simulink model "Disconnections_ETR07"  (R2017b)
settings: Solver=FixedStepAuto  StartTime=0.0  StopTime=10.0  RelTol=1e-3
libraries: simulink x7
settings Model: Creator=cspt  LastModifiedBy=cspt
settings RTWCC: SystemTargetFile=irt.tlc  TemplateMakefile=irt_default_tmf  Description=INTECRIO Real-Time Target
settings STFCustomTargetCC: TargetLangStandard=C99 (ISO)  UtilityFuncGeneration=Shared location  SystemTargetFile=irt.tlc
settings GRTTargetCC: UtilityFuncGeneration=Shared location  ParMdlRefBuildCompliant=off  CompOptLevelCompliant=off  ConcurrentExecutionCompliant=off  CombineOutputUpdateFcns=off  MatFileLogging=off  CPPClassGenCompliant=off  GRTInterface=on  UseToolchainInfoCompliant=off  GenerateASAP2=on

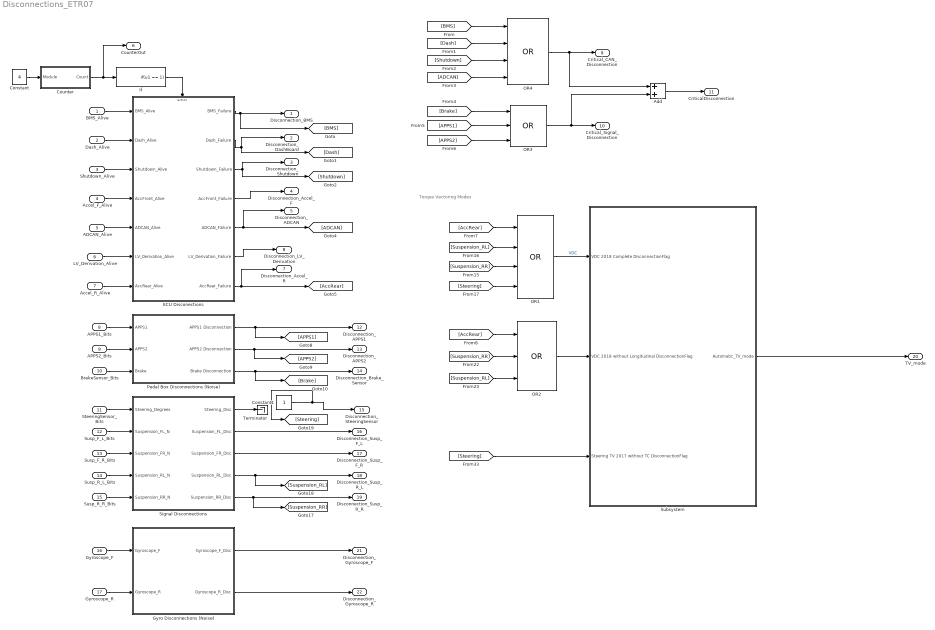
== system Disconnections_ETR07 ==
  note: Torque Vectoring Modes
  BMS_Alive : Inport
  Dash_Alive : Inport  Port=2
  Shutdown_Alive : Inport  Port=3
  Accel_F_Alive : Inport  Port=4
  ADCAN_Alive : Inport  Port=5
  LV_Derivation_Alive : Inport  Port=6
  Accel_R_Alive : Inport  Port=7
  APPS1_Bits : Inport  Port=8
  APPS2_Bits : Inport  Port=9
  BrakeSensor_Bits : Inport  Port=10
  SteeringSensor_Bits : Inport  Port=11
  Susp_F_L_Bits : Inport  Port=12
  Susp_F_R_Bits : Inport  Port=13
  Susp_R_L_Bits : Inport  Port=14
  Susp_R_R_Bits : Inport  Port=15
  Gyroscope_F : Inport  Port=16
  Gyroscope_R : Inport  Port=17
  Add : Sum
  Constant : Constant  Value=4
  Constant1 : Constant
  Counter : Subsystem
  ECU Disconections : Subsystem
  Gyro Disconnections (Noise) : Subsystem
  If : If  IfExpression=u1 == 1  ShowElse=off
  OR1 : Logic  Operator=OR  Inputs=4  AllPortsSameDT=off  OutDataTypeStr=boolean
  OR2 : Logic  Operator=OR  Inputs=3  AllPortsSameDT=off  OutDataTypeStr=boolean
  OR3 : Logic  Operator=OR  Inputs=3  AllPortsSameDT=off  OutDataTypeStr=boolean
  OR4 : Logic  Operator=OR  Inputs=4  AllPortsSameDT=off  OutDataTypeStr=boolean
  Pedal Box Disconnections (Noise) : Subsystem
  Signal Disconnections : Subsystem
  Subsystem : Subsystem
  Terminator : Terminator
  Disconnection_BMS : Outport
  Disconnection_DashBoard : Outport  Port=2
  Disconnection_Shutdown : Outport  Port=3
  Disconnection_Accel_F : Outport  Port=4
  Disconnection_ADCAN : Outport  Port=5
  CounterOut : Outport  Port=6
  Disconnection_Accel_R : Outport  Port=7
  Disconnection_LV_Derivation : Outport  Port=8
  Critical_CAN_Disconnection : Outport  Port=9
  Critical_Signal_Disconnection : Outport  Port=10
  CriticalDisconnection : Outport  Port=11
  Disconnection_APPS1 : Outport  Port=12
  Disconnection_APPS2 : Outport  Port=13
  Disconnection_Brake_Sensor : Outport  Port=14
  Disconnection_SteeringSensor : Outport  Port=15
  Disconnection_Susp_F_L : Outport  Port=16
  Disconnection_Susp_F_R : Outport  Port=17
  Disconnection_Susp_R_L : Outport  Port=18
  Disconnection_Susp_R_R : Outport  Port=19
  TV_mode : Outport  Port=20
  Disconnection_Gyroscope_F : Outport  Port=21
  Disconnection_Gyroscope_R : Outport  Port=22
  wires:
  LV_Derivation_Alive/1 -> ECU Disconections/6(LV_Derivation_Alive)
  Accel_R_Alive/1 -> ECU Disconections/7(AccRear_Alive)
  ECU Disconections/7(AccRear_Failure) -> [AccRear], Disconnection_Accel_R/1
  ECU Disconections/5(ADCAN_Failure) -> Disconnection_ADCAN/1, [ADCAN]
  ECU Disconections/1(BMS_Failure) -> Disconnection_BMS/1, [BMS]
  Dash_Alive/1 -> ECU Disconections/2(Dash_Alive)
  ECU Disconections/4(AccFront_Failure) -> Disconnection_Accel_F/1
  Counter/1(Count) -> CounterOut/1, If/1
  ECU Disconections/6(LV_Derivation_Failure) -> Disconnection_LV_Derivation/1
  Accel_F_Alive/1 -> ECU Disconections/4(AccFront_Alive)
  BMS_Alive/1 -> ECU Disconections/1(BMS_Alive)
  Constant/1 -> Counter/1(Module)
  ECU Disconections/2(Dash_Failure) -> Disconnection_DashBoard/1, [Dash]
  Shutdown_Alive/1 -> ECU Disconections/3(Shutdown_Alive)
  If/1 -> ECU Disconections/Action
  ECU Disconections/3(Shutdown_Failure) -> [Shutdown], Disconnection_Shutdown/1
  ADCAN_Alive/1 -> ECU Disconections/5(ADCAN_Alive)
  [Shutdown] -> OR4/3
  [Dash] -> OR4/2
  [BMS] -> OR4/1
  [ADCAN] -> OR4/4
  [Brake] -> OR3/1
  [APPS1] -> OR3/2
  OR3/1 -> Add/2, Critical_Signal_Disconnection/1
  [APPS2] -> OR3/3
  Add/1 -> CriticalDisconnection/1
  OR4/1 -> Add/1, Critical_CAN_Disconnection/1
  Pedal Box Disconnections (Noise)/2(APPS2 Disconnection) -> Disconnection_APPS2/1, [APPS2]
  Pedal Box Disconnections (Noise)/3(Brake Disconnection) -> Disconnection_Brake_Sensor/1, [Brake]
  APPS2_Bits/1 -> Pedal Box Disconnections (Noise)/2(APPS2)
  BrakeSensor_Bits/1 -> Pedal Box Disconnections (Noise)/3(Brake)
  Pedal Box Disconnections (Noise)/1(APPS1 Disconnection) -> [APPS1], Disconnection_APPS1/1
  APPS1_Bits/1 -> Pedal Box Disconnections (Noise)/1(APPS1)
  Signal Disconnections/2(Suspension_FL_Disc) -> Disconnection_Susp_F_L/1
  Susp_R_L_Bits/1 -> Signal Disconnections/4(Suspension_RL_N)
  Signal Disconnections/4(Suspension_RL_Disc) -> Disconnection_Susp_R_L/1, [Suspension_RL]
  Signal Disconnections/5(Suspension_RR_Disc) -> Disconnection_Susp_R_R/1, [Suspension_RR]
  Susp_R_R_Bits/1 -> Signal Disconnections/5(Suspension_RR_N)
  Signal Disconnections/3(Suspension_FR_Disc) -> Disconnection_Susp_F_R/1
  Susp_F_R_Bits/1 -> Signal Disconnections/3(Suspension_FR_N)
  Susp_F_L_Bits/1 -> Signal Disconnections/2(Suspension_FL_N)
  SteeringSensor_Bits/1 -> Signal Disconnections/1(Steering_Degrees)
  [Steering] -> Subsystem/3(Steering TV 2017 without TC DisconnectionFlag)
  OR1/1 -> Subsystem/1(VDC 2018 Complete DisconnectionFlag)  "VDC"
  [Suspension_RR] -> OR2/2
  OR2/1 -> Subsystem/2(VDC 2018 without Longitudinal DisconnectionFlag)
  Subsystem/1(Automatic_TV_mode) -> TV_mode/1
  [Suspension_RL] -> OR2/3
  [AccRear] -> OR2/1
  [AccRear] -> OR1/1
  Gyro Disconnections (Noise)/2(Gyroscope_R_Disc) -> Disconnection_Gyroscope_R/1
  Gyro Disconnections (Noise)/1(Gyroscope_F_Disc) -> Disconnection_Gyroscope_F/1
  Gyroscope_R/1 -> Gyro Disconnections (Noise)/2(Gyroscope_R)
  Gyroscope_F/1 -> Gyro Disconnections (Noise)/1(Gyroscope_F)
  [Suspension_RL] -> OR1/2
  [Suspension_RR] -> OR1/3
  [Steering] -> OR1/4
  Signal Disconnections/1(Steering_Disc) -> Terminator/1
  Constant1/1 -> [Steering], Disconnection_SteeringSensor/1

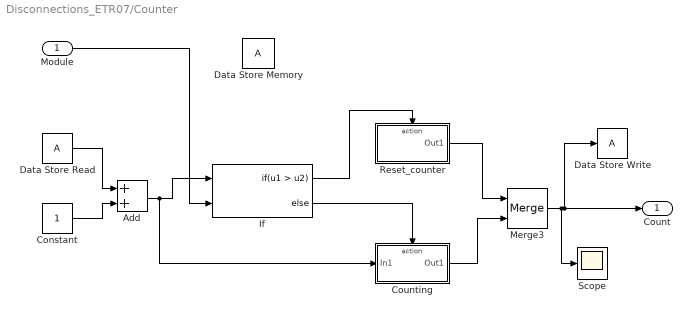
== system Disconnections_ETR07/Counter ==
  Module : Inport
  Add : Sum
  Constant : Constant
  Counting : Subsystem  TreatAsAtomicUnit=on
  Data Store Memory : DataStoreMemory  ReadBeforeWriteMsg=warning  WriteAfterWriteMsg=warning  WriteAfterReadMsg=warning  ShowAdditionalParam=off
  Data Store Read : DataStoreRead
  Data Store Write : DataStoreWrite
  If : If  NumInputs=2  IfExpression=u1 > u2
  Merge3 : Merge
  Reset_counter : Subsystem  TreatAsAtomicUnit=on
  Scope : Scope
  Count : Outport
  wires:
  Data Store Read/1 -> Add/1
  Constant/1 -> Add/2
  Add/1 -> If/1, Counting/1(In1)
  If/1 -> Reset_counter/Action
  If/2 -> Counting/Action
  Reset_counter/1(Out1) -> Merge3/1
  Counting/1(Out1) -> Merge3/2
  Module/1 -> If/2
  Merge3/1 -> Scope/1, Data Store Write/1, Count/1

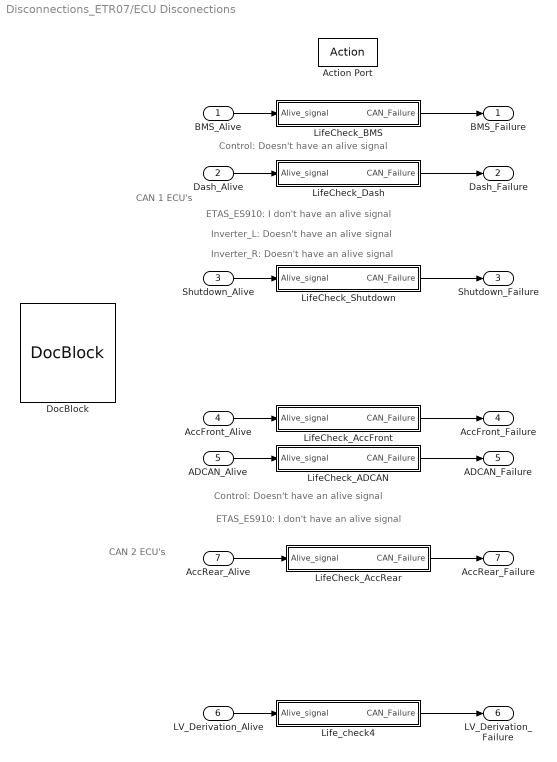
== system Disconnections_ETR07/ECU Disconections ==
  note: ETAS_ES910: I don't have an alive signal
  note: Control: Doesn't have an alive signal
  note: CAN 1
      | ECU's
  note: Inverter_L: Doesn't have an alive signal
  note: Inverter_R: Doesn't have an alive signal
  note: Control: Doesn't have an alive signal
  note: ETAS_ES910: I don't have an alive signal
  note: CAN 2
      | ECU's
  BMS_Alive : Inport
  Dash_Alive : Inport  Port=2
  Shutdown_Alive : Inport  Port=3
  AccFront_Alive : Inport  Port=4
  ADCAN_Alive : Inport  Port=5
  LV_Derivation_Alive : Inport  Port=6
  AccRear_Alive : Inport  Port=7
  Action Port : ActionPort  ActionType=then
  DocBlock : simulink/Model-Wide Utilities/DocBlock  DocumentType=Text
      content=|
      | The Alive signal is sent and updated every 4 synchronisms (25ms x 4 = 100ms).
      |
      | This is a Network Management Module. It takes all the alive signals of the ECU's and check if they are "alive".
      | All the ECU's for each CAN database have been extracted and listed. Some ECU's do not have an alive signal.
      |
      | Each LifeCheck generates a signal that indicate if the ECU has been disconnected.
      | OK -> 0
      | Disconnected -> 1
  LifeCheck_ADCAN : Subsystem
  LifeCheck_AccFront : Subsystem
  LifeCheck_AccRear : Subsystem
  LifeCheck_BMS : Subsystem
  LifeCheck_Dash : Subsystem
  LifeCheck_Shutdown : Subsystem
  Life_check4 : Subsystem
  BMS_Failure : Outport
  Dash_Failure : Outport  Port=2
  Shutdown_Failure : Outport  Port=3
  AccFront_Failure : Outport  Port=4
  ADCAN_Failure : Outport  Port=5
  LV_Derivation_Failure : Outport  Port=6
  AccRear_Failure : Outport  Port=7
  wires:
  Life_check4/1(CAN_Failure) -> LV_Derivation_Failure/1
  LV_Derivation_Alive/1 -> Life_check4/1(Alive_signal)
  LifeCheck_AccFront/1(CAN_Failure) -> AccFront_Failure/1
  LifeCheck_Shutdown/1(CAN_Failure) -> Shutdown_Failure/1
  LifeCheck_Dash/1(CAN_Failure) -> Dash_Failure/1
  Dash_Alive/1 -> LifeCheck_Dash/1(Alive_signal)
  LifeCheck_ADCAN/1(CAN_Failure) -> ADCAN_Failure/1
  LifeCheck_BMS/1(CAN_Failure) -> BMS_Failure/1
  AccFront_Alive/1 -> LifeCheck_AccFront/1(Alive_signal)
  BMS_Alive/1 -> LifeCheck_BMS/1(Alive_signal)
  ADCAN_Alive/1 -> LifeCheck_ADCAN/1(Alive_signal)
  Shutdown_Alive/1 -> LifeCheck_Shutdown/1(Alive_signal)
  LifeCheck_AccRear/1(CAN_Failure) -> AccRear_Failure/1
  AccRear_Alive/1 -> LifeCheck_AccRear/1(Alive_signal)

== system Disconnections_ETR07/Gyro Disconnections (Noise) ==
  Gyroscope_F : Inport
  Gyroscope_R : Inport  Port=2
  Life_check6 : Subsystem
  Life_check8 : Subsystem
  Gyroscope_F_Disc : Outport
  Gyroscope_R_Disc : Outport  Port=2
  wires:
  Gyroscope_F/1 -> Life_check6/1(Signal)
  Life_check8/1(Disconnect_Fail) -> Gyroscope_R_Disc/1
  Gyroscope_R/1 -> Life_check8/1(Signal)
  Life_check6/1(Disconnect_Fail) -> Gyroscope_F_Disc/1

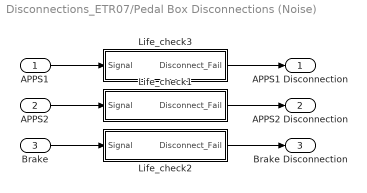
== system Disconnections_ETR07/Pedal Box Disconnections (Noise) ==
  APPS1 : Inport
  APPS2 : Inport  Port=2
  Brake : Inport  Port=3
  Life_check1 : Subsystem
  Life_check2 : Subsystem
  Life_check3 : Subsystem
  APPS1 Disconnection : Outport
  APPS2 Disconnection : Outport  Port=2
  Brake Disconnection : Outport  Port=3
  wires:
  Brake/1 -> Life_check2/1(Signal)
  APPS2/1 -> Life_check1/1(Signal)
  APPS1/1 -> Life_check3/1(Signal)
  Life_check3/1(Disconnect_Fail) -> APPS1 Disconnection/1
  Life_check1/1(Disconnect_Fail) -> APPS2 Disconnection/1
  Life_check2/1(Disconnect_Fail) -> Brake Disconnection/1

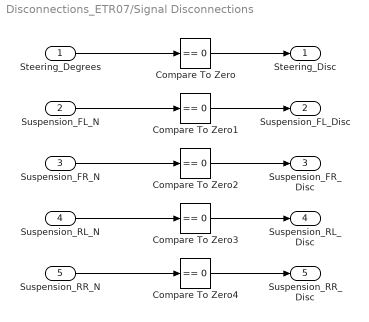
== system Disconnections_ETR07/Signal Disconnections ==
  Steering_Degrees : Inport
  Suspension_FL_N : Inport  Port=2
  Suspension_FR_N : Inport  Port=3
  Suspension_RL_N : Inport  Port=4
  Suspension_RR_N : Inport  Port=5
  Compare To Zero{,1..4} (5 alike) : simulink/Logic and Bit Operations/Compare To Zero  relop===  OutDataTypeStr=uint8
  Steering_Disc : Outport
  Suspension_FL_Disc : Outport  Port=2
  Suspension_FR_Disc : Outport  Port=3
  Suspension_RL_Disc : Outport  Port=4
  Suspension_RR_Disc : Outport  Port=5
  wires:
  Compare To Zero2/1 -> Suspension_FR_Disc/1
  Suspension_FR_N/1 -> Compare To Zero2/1
  Compare To Zero3/1 -> Suspension_RL_Disc/1
  Compare To Zero1/1 -> Suspension_FL_Disc/1
  Suspension_RR_N/1 -> Compare To Zero4/1
  Suspension_FL_N/1 -> Compare To Zero1/1
  Suspension_RL_N/1 -> Compare To Zero3/1
  Compare To Zero/1 -> Steering_Disc/1
  Steering_Degrees/1 -> Compare To Zero/1
  Compare To Zero4/1 -> Suspension_RR_Disc/1

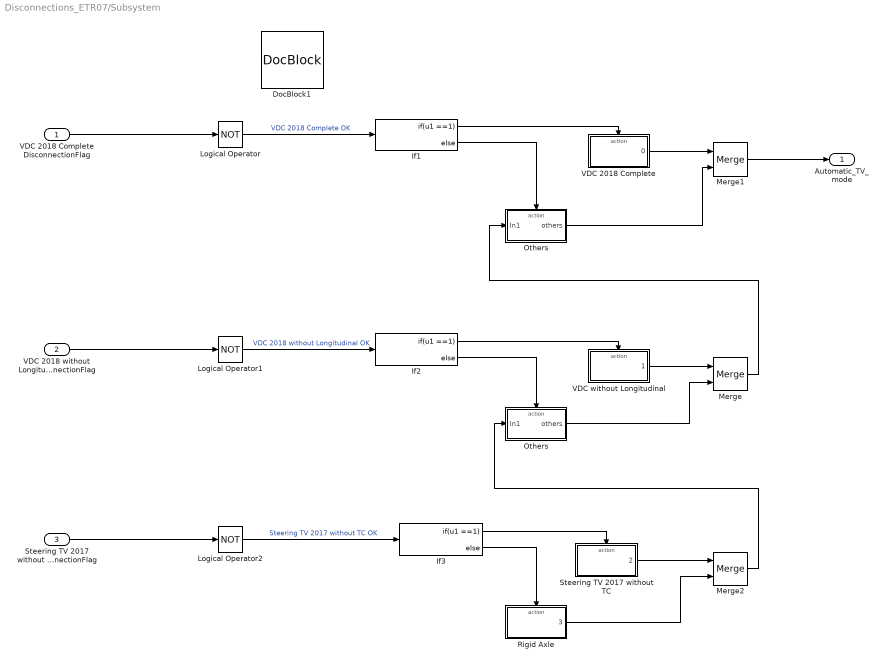
== system Disconnections_ETR07/Subsystem ==
  VDC 2018 Complete DisconnectionFlag : Inport
  VDC 2018 without Longitudinal DisconnectionFlag : Inport  Port=2
  Steering TV 2017 without TC DisconnectionFlag : Inport  Port=3
  DocBlock1 : simulink/Model-Wide Utilities/DocBlock  DocumentType=Text
      content=|
      | Checking for APPS, Brake etc... would be redundant since they are critical disconnections and the car will enter to a stop state
  If1 : If  IfExpression=u1 ==1
  If2 : If  IfExpression=u1 ==1
  If3 : If  IfExpression=u1 ==1
  Logical Operator : Logic  Operator=NOT  AllPortsSameDT=off  OutDataTypeStr=boolean
  Logical Operator1 : Logic  Operator=NOT  AllPortsSameDT=off  OutDataTypeStr=boolean
  Logical Operator2 : Logic  Operator=NOT  AllPortsSameDT=off  OutDataTypeStr=boolean
  Merge : Merge
  Merge1 : Merge
  Merge2 : Merge
  Others : Subsystem  TreatAsAtomicUnit=on
  "Others " : Subsystem  TreatAsAtomicUnit=on
  Rigid Axle : Subsystem  TreatAsAtomicUnit=on
  Steering TV 2017 without TC : Subsystem  TreatAsAtomicUnit=on
  VDC 2018 Complete : Subsystem  TreatAsAtomicUnit=on
  "VDC without Longitudinal " : Subsystem  TreatAsAtomicUnit=on
  Automatic_TV_mode : Outport
  wires:
  VDC 2018 Complete DisconnectionFlag/1 -> Logical Operator/1
  Logical Operator2/1 -> If3/1  "Steering TV 2017 without TC OK"
  "Others "/1(others) -> Merge/2
  If1/2 -> Others/Action
  "VDC without Longitudinal "/1(1) -> Merge/1
  VDC 2018 without Longitudinal DisconnectionFlag/1 -> Logical Operator1/1
  Logical Operator1/1 -> If2/1  "VDC 2018 without Longitudinal OK"
  Steering TV 2017 without TC DisconnectionFlag/1 -> Logical Operator2/1
  If1/1 -> VDC 2018 Complete/Action
  Logical Operator/1 -> If1/1  "VDC 2018 Complete OK"
  If2/2 -> "Others "/Action
  If2/1 -> "VDC without Longitudinal "/Action
  Merge/1 -> Others/1(In1)
  VDC 2018 Complete/1(0) -> Merge1/1
  Rigid Axle/1(3) -> Merge2/2
  Merge2/1 -> "Others "/1(In1)
  Merge1/1 -> Automatic_TV_mode/1
  If3/2 -> Rigid Axle/Action
  If3/1 -> Steering TV 2017 without TC/Action
  Steering TV 2017 without TC/1(2) -> Merge2/1
  Others/1(others) -> Merge1/2

== system Disconnections_ETR07/Counter/Counting ==
  In1 : Inport
  Action Port : ActionPort  ActionType=else
  Out1 : Outport
  wires:
  In1/1 -> Out1/1

== system Disconnections_ETR07/Counter/Reset_counter ==
  Action Port : ActionPort  ActionType=then
  Constant : Constant
  Out1 : Outport
  wires:
  Constant/1 -> Out1/1

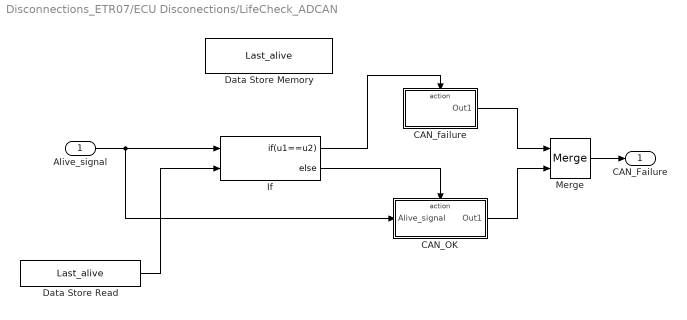
== system Disconnections_ETR07/ECU Disconections/LifeCheck_ADCAN ==
  Alive_signal : Inport
  CAN_OK : Subsystem  TreatAsAtomicUnit=on
  CAN_failure : Subsystem  TreatAsAtomicUnit=on
  Data Store Memory : DataStoreMemory  DataStoreName=Last_alive  ReadBeforeWriteMsg=warning  WriteAfterWriteMsg=warning  WriteAfterReadMsg=warning  ShowAdditionalParam=off
  Data Store Read : DataStoreRead  DataStoreName=Last_alive
  If : If  NumInputs=2  IfExpression=u1==u2
  Merge : Merge
  CAN_Failure : Outport
  wires:
  Data Store Read/1 -> If/2
  If/1 -> CAN_failure/Action
  If/2 -> CAN_OK/Action
  CAN_failure/1(Out1) -> Merge/1
  CAN_OK/1(Out1) -> Merge/2
  Merge/1 -> CAN_Failure/1
  Alive_signal/1 -> CAN_OK/1(Alive_signal), If/1

== system Disconnections_ETR07/ECU Disconections/LifeCheck_AccFront ==
  Alive_signal : Inport
  CAN_OK : Subsystem  TreatAsAtomicUnit=on
  CAN_failure : Subsystem  TreatAsAtomicUnit=on
  Data Store Memory : DataStoreMemory  DataStoreName=Last_alive  ReadBeforeWriteMsg=warning  WriteAfterWriteMsg=warning  WriteAfterReadMsg=warning  ShowAdditionalParam=off
  Data Store Read : DataStoreRead  DataStoreName=Last_alive
  If : If  NumInputs=2  IfExpression=u1==u2
  Merge : Merge
  CAN_Failure : Outport
  wires:
  Data Store Read/1 -> If/2
  If/1 -> CAN_failure/Action
  If/2 -> CAN_OK/Action
  CAN_failure/1(Out1) -> Merge/1
  CAN_OK/1(Out1) -> Merge/2
  Merge/1 -> CAN_Failure/1
  Alive_signal/1 -> CAN_OK/1(Alive_signal), If/1

== system Disconnections_ETR07/ECU Disconections/LifeCheck_AccRear ==
  Alive_signal : Inport
  CAN_OK : Subsystem  TreatAsAtomicUnit=on
  CAN_failure : Subsystem  TreatAsAtomicUnit=on
  Data Store Memory : DataStoreMemory  DataStoreName=Last_alive  ReadBeforeWriteMsg=warning  WriteAfterWriteMsg=warning  WriteAfterReadMsg=warning  ShowAdditionalParam=off
  Data Store Read : DataStoreRead  DataStoreName=Last_alive
  If : If  NumInputs=2  IfExpression=u1==u2
  Merge : Merge
  CAN_Failure : Outport
  wires:
  Data Store Read/1 -> If/2
  If/1 -> CAN_failure/Action
  If/2 -> CAN_OK/Action
  CAN_failure/1(Out1) -> Merge/1
  CAN_OK/1(Out1) -> Merge/2
  Merge/1 -> CAN_Failure/1
  Alive_signal/1 -> CAN_OK/1(Alive_signal), If/1

== system Disconnections_ETR07/ECU Disconections/LifeCheck_BMS ==
  Alive_signal : Inport
  CAN_OK : Subsystem  TreatAsAtomicUnit=on
  CAN_failure : Subsystem  TreatAsAtomicUnit=on
  Data Store Memory : DataStoreMemory  DataStoreName=Last_alive  ReadBeforeWriteMsg=warning  WriteAfterWriteMsg=warning  WriteAfterReadMsg=warning  ShowAdditionalParam=off
  Data Store Read : DataStoreRead  DataStoreName=Last_alive
  If : If  NumInputs=2  IfExpression=u1==u2
  Merge : Merge
  CAN_Failure : Outport
  wires:
  Data Store Read/1 -> If/2
  If/1 -> CAN_failure/Action
  If/2 -> CAN_OK/Action
  CAN_failure/1(Out1) -> Merge/1
  CAN_OK/1(Out1) -> Merge/2
  Merge/1 -> CAN_Failure/1
  Alive_signal/1 -> CAN_OK/1(Alive_signal), If/1

== system Disconnections_ETR07/ECU Disconections/LifeCheck_Dash ==
  Alive_signal : Inport
  CAN_OK : Subsystem  TreatAsAtomicUnit=on
  CAN_failure : Subsystem  TreatAsAtomicUnit=on
  Data Store Memory : DataStoreMemory  DataStoreName=Last_alive  ReadBeforeWriteMsg=warning  WriteAfterWriteMsg=warning  WriteAfterReadMsg=warning  ShowAdditionalParam=off
  Data Store Read : DataStoreRead  DataStoreName=Last_alive
  If : If  NumInputs=2  IfExpression=u1==u2
  Merge : Merge
  CAN_Failure : Outport
  wires:
  Data Store Read/1 -> If/2
  If/1 -> CAN_failure/Action
  If/2 -> CAN_OK/Action
  CAN_failure/1(Out1) -> Merge/1
  CAN_OK/1(Out1) -> Merge/2
  Merge/1 -> CAN_Failure/1
  Alive_signal/1 -> CAN_OK/1(Alive_signal), If/1

== system Disconnections_ETR07/ECU Disconections/LifeCheck_Shutdown ==
  Alive_signal : Inport
  CAN_OK : Subsystem  TreatAsAtomicUnit=on
  CAN_failure : Subsystem  TreatAsAtomicUnit=on
  Data Store Memory : DataStoreMemory  DataStoreName=Last_alive  ReadBeforeWriteMsg=warning  WriteAfterWriteMsg=warning  WriteAfterReadMsg=warning  ShowAdditionalParam=off
  Data Store Read : DataStoreRead  DataStoreName=Last_alive
  If : If  NumInputs=2  IfExpression=u1==u2
  Merge : Merge
  CAN_Failure : Outport
  wires:
  Data Store Read/1 -> If/2
  If/1 -> CAN_failure/Action
  If/2 -> CAN_OK/Action
  CAN_failure/1(Out1) -> Merge/1
  CAN_OK/1(Out1) -> Merge/2
  Merge/1 -> CAN_Failure/1
  Alive_signal/1 -> CAN_OK/1(Alive_signal), If/1

== system Disconnections_ETR07/ECU Disconections/Life_check4 ==
  Alive_signal : Inport
  CAN_OK : Subsystem  TreatAsAtomicUnit=on
  CAN_failure : Subsystem  TreatAsAtomicUnit=on
  Data Store Memory : DataStoreMemory  DataStoreName=Last_alive  ReadBeforeWriteMsg=warning  WriteAfterWriteMsg=warning  WriteAfterReadMsg=warning  ShowAdditionalParam=off
  Data Store Read : DataStoreRead  DataStoreName=Last_alive
  If : If  NumInputs=2  IfExpression=u1==u2
  Merge : Merge
  CAN_Failure : Outport
  wires:
  Data Store Read/1 -> If/2
  If/1 -> CAN_failure/Action
  If/2 -> CAN_OK/Action
  CAN_failure/1(Out1) -> Merge/1
  CAN_OK/1(Out1) -> Merge/2
  Merge/1 -> CAN_Failure/1
  Alive_signal/1 -> CAN_OK/1(Alive_signal), If/1

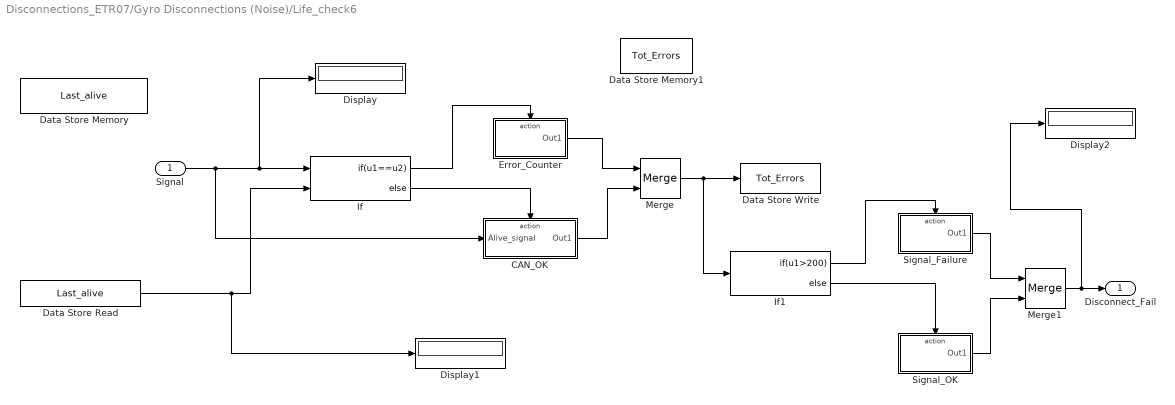
== system Disconnections_ETR07/Gyro Disconnections (Noise)/Life_check6 ==
  Signal : Inport
  CAN_OK : Subsystem  TreatAsAtomicUnit=on
  Data Store Memory : DataStoreMemory  DataStoreName=Last_alive  ReadBeforeWriteMsg=warning  WriteAfterWriteMsg=warning  WriteAfterReadMsg=warning  ShowAdditionalParam=off
  Data Store Memory1 : DataStoreMemory  DataStoreName=Tot_Errors  ReadBeforeWriteMsg=warning  WriteAfterWriteMsg=warning  WriteAfterReadMsg=warning  ShowAdditionalParam=off
  Data Store Read : DataStoreRead  DataStoreName=Last_alive
  Data Store Write : DataStoreWrite  DataStoreName=Tot_Errors
  Display : Display
  Display1 : Display
  Display2 : Display
  Error_Counter : Subsystem  TreatAsAtomicUnit=on
  If : If  NumInputs=2  IfExpression=u1==u2
  If1 : If  IfExpression=u1>200
  Merge : Merge
  Merge1 : Merge
  Signal_Failure : Subsystem  TreatAsAtomicUnit=on
  Signal_OK : Subsystem  TreatAsAtomicUnit=on
  Disconnect_Fail : Outport
  wires:
  Data Store Read/1 -> Display1/1, If/2
  If/2 -> CAN_OK/Action
  CAN_OK/1(Out1) -> Merge/2
  Merge/1 -> If1/1, Data Store Write/1
  Signal/1 -> CAN_OK/1(Alive_signal), Display/1, If/1
  If/1 -> Error_Counter/Action
  Error_Counter/1(Out1) -> Merge/1
  If1/1 -> Signal_Failure/Action
  If1/2 -> Signal_OK/Action
  Signal_Failure/1(Out1) -> Merge1/1
  Signal_OK/1(Out1) -> Merge1/2
  Merge1/1 -> Display2/1, Disconnect_Fail/1

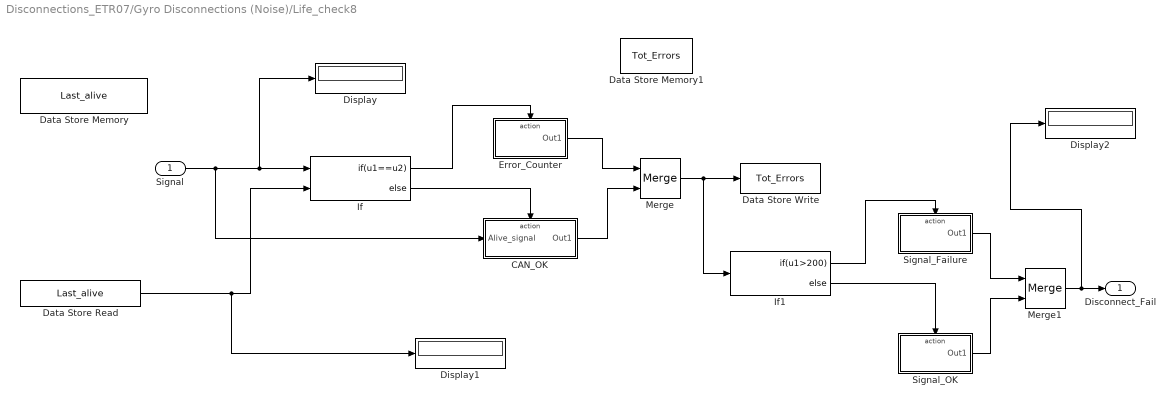
== system Disconnections_ETR07/Gyro Disconnections (Noise)/Life_check8 ==
  Signal : Inport
  CAN_OK : Subsystem  TreatAsAtomicUnit=on
  Data Store Memory : DataStoreMemory  DataStoreName=Last_alive  ReadBeforeWriteMsg=warning  WriteAfterWriteMsg=warning  WriteAfterReadMsg=warning  ShowAdditionalParam=off
  Data Store Memory1 : DataStoreMemory  DataStoreName=Tot_Errors  ReadBeforeWriteMsg=warning  WriteAfterWriteMsg=warning  WriteAfterReadMsg=warning  ShowAdditionalParam=off
  Data Store Read : DataStoreRead  DataStoreName=Last_alive
  Data Store Write : DataStoreWrite  DataStoreName=Tot_Errors
  Display : Display
  Display1 : Display
  Display2 : Display
  Error_Counter : Subsystem  TreatAsAtomicUnit=on
  If : If  NumInputs=2  IfExpression=u1==u2
  If1 : If  IfExpression=u1>200
  Merge : Merge
  Merge1 : Merge
  Signal_Failure : Subsystem  TreatAsAtomicUnit=on
  Signal_OK : Subsystem  TreatAsAtomicUnit=on
  Disconnect_Fail : Outport
  wires:
  Data Store Read/1 -> Display1/1, If/2
  If/2 -> CAN_OK/Action
  CAN_OK/1(Out1) -> Merge/2
  Merge/1 -> If1/1, Data Store Write/1
  Signal/1 -> CAN_OK/1(Alive_signal), Display/1, If/1
  If/1 -> Error_Counter/Action
  Error_Counter/1(Out1) -> Merge/1
  If1/1 -> Signal_Failure/Action
  If1/2 -> Signal_OK/Action
  Signal_Failure/1(Out1) -> Merge1/1
  Signal_OK/1(Out1) -> Merge1/2
  Merge1/1 -> Display2/1, Disconnect_Fail/1

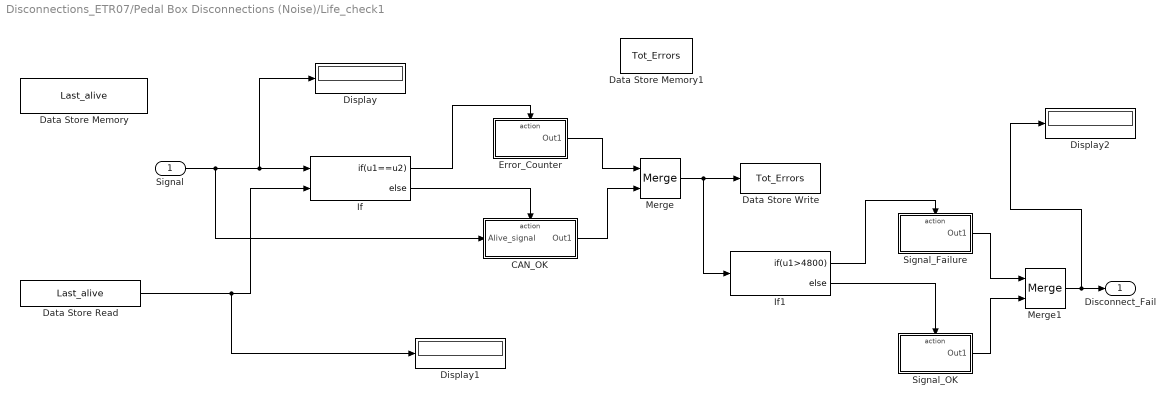
== system Disconnections_ETR07/Pedal Box Disconnections (Noise)/Life_check1 ==
  Signal : Inport
  CAN_OK : Subsystem  TreatAsAtomicUnit=on
  Data Store Memory : DataStoreMemory  DataStoreName=Last_alive  ReadBeforeWriteMsg=warning  WriteAfterWriteMsg=warning  WriteAfterReadMsg=warning  ShowAdditionalParam=off
  Data Store Memory1 : DataStoreMemory  DataStoreName=Tot_Errors  ReadBeforeWriteMsg=warning  WriteAfterWriteMsg=warning  WriteAfterReadMsg=warning  ShowAdditionalParam=off
  Data Store Read : DataStoreRead  DataStoreName=Last_alive
  Data Store Write : DataStoreWrite  DataStoreName=Tot_Errors
  Display : Display
  Display1 : Display
  Display2 : Display
  Error_Counter : Subsystem  TreatAsAtomicUnit=on
  If : If  NumInputs=2  IfExpression=u1==u2
  If1 : If  IfExpression=u1>4800
  Merge : Merge
  Merge1 : Merge
  Signal_Failure : Subsystem  TreatAsAtomicUnit=on
  Signal_OK : Subsystem  TreatAsAtomicUnit=on
  Disconnect_Fail : Outport
  wires:
  Data Store Read/1 -> Display1/1, If/2
  If/2 -> CAN_OK/Action
  CAN_OK/1(Out1) -> Merge/2
  Merge/1 -> If1/1, Data Store Write/1
  Signal/1 -> CAN_OK/1(Alive_signal), Display/1, If/1
  If/1 -> Error_Counter/Action
  Error_Counter/1(Out1) -> Merge/1
  If1/1 -> Signal_Failure/Action
  If1/2 -> Signal_OK/Action
  Signal_Failure/1(Out1) -> Merge1/1
  Signal_OK/1(Out1) -> Merge1/2
  Merge1/1 -> Display2/1, Disconnect_Fail/1

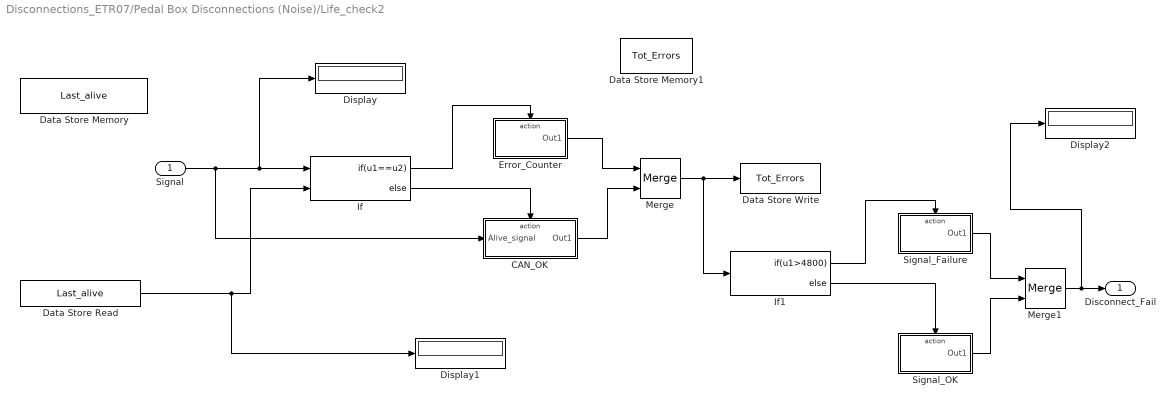
== system Disconnections_ETR07/Pedal Box Disconnections (Noise)/Life_check2 ==
  Signal : Inport
  CAN_OK : Subsystem  TreatAsAtomicUnit=on
  Data Store Memory : DataStoreMemory  DataStoreName=Last_alive  ReadBeforeWriteMsg=warning  WriteAfterWriteMsg=warning  WriteAfterReadMsg=warning  ShowAdditionalParam=off
  Data Store Memory1 : DataStoreMemory  DataStoreName=Tot_Errors  ReadBeforeWriteMsg=warning  WriteAfterWriteMsg=warning  WriteAfterReadMsg=warning  ShowAdditionalParam=off
  Data Store Read : DataStoreRead  DataStoreName=Last_alive
  Data Store Write : DataStoreWrite  DataStoreName=Tot_Errors
  Display : Display
  Display1 : Display
  Display2 : Display
  Error_Counter : Subsystem  TreatAsAtomicUnit=on
  If : If  NumInputs=2  IfExpression=u1==u2
  If1 : If  IfExpression=u1>4800
  Merge : Merge
  Merge1 : Merge
  Signal_Failure : Subsystem  TreatAsAtomicUnit=on
  Signal_OK : Subsystem  TreatAsAtomicUnit=on
  Disconnect_Fail : Outport
  wires:
  Data Store Read/1 -> Display1/1, If/2
  If/2 -> CAN_OK/Action
  CAN_OK/1(Out1) -> Merge/2
  Merge/1 -> If1/1, Data Store Write/1
  Signal/1 -> CAN_OK/1(Alive_signal), Display/1, If/1
  If/1 -> Error_Counter/Action
  Error_Counter/1(Out1) -> Merge/1
  If1/1 -> Signal_Failure/Action
  If1/2 -> Signal_OK/Action
  Signal_Failure/1(Out1) -> Merge1/1
  Signal_OK/1(Out1) -> Merge1/2
  Merge1/1 -> Display2/1, Disconnect_Fail/1

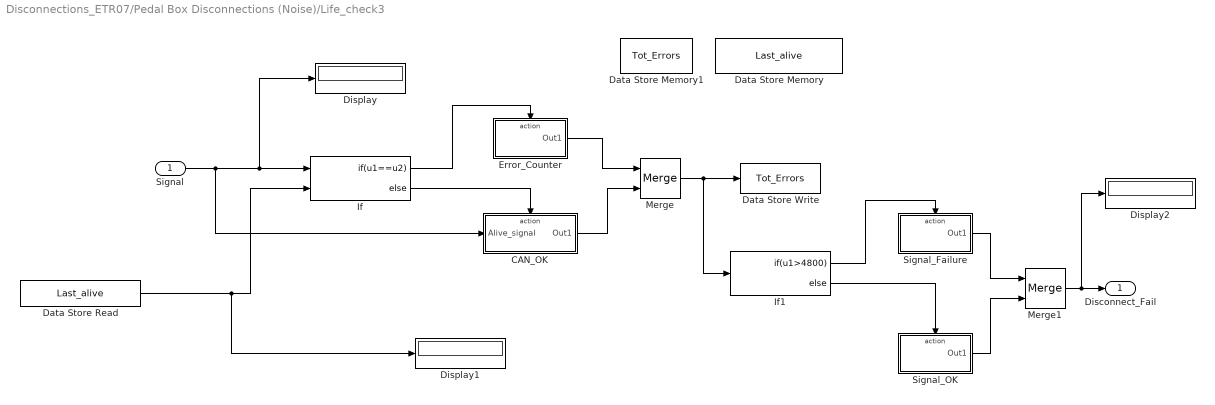
== system Disconnections_ETR07/Pedal Box Disconnections (Noise)/Life_check3 ==
  Signal : Inport
  CAN_OK : Subsystem  TreatAsAtomicUnit=on
  Data Store Memory : DataStoreMemory  DataStoreName=Last_alive  ReadBeforeWriteMsg=warning  WriteAfterWriteMsg=warning  WriteAfterReadMsg=warning  ShowAdditionalParam=off
  Data Store Memory1 : DataStoreMemory  DataStoreName=Tot_Errors  ReadBeforeWriteMsg=warning  WriteAfterWriteMsg=warning  WriteAfterReadMsg=warning  ShowAdditionalParam=off
  Data Store Read : DataStoreRead  DataStoreName=Last_alive
  Data Store Write : DataStoreWrite  DataStoreName=Tot_Errors
  Display : Display
  Display1 : Display
  Display2 : Display
  Error_Counter : Subsystem  TreatAsAtomicUnit=on
  If : If  NumInputs=2  IfExpression=u1==u2
  If1 : If  IfExpression=u1>4800
  Merge : Merge
  Merge1 : Merge
  Signal_Failure : Subsystem  TreatAsAtomicUnit=on
  Signal_OK : Subsystem  TreatAsAtomicUnit=on
  Disconnect_Fail : Outport
  wires:
  Data Store Read/1 -> Display1/1, If/2
  If/2 -> CAN_OK/Action
  CAN_OK/1(Out1) -> Merge/2
  Merge/1 -> If1/1, Data Store Write/1
  Signal/1 -> CAN_OK/1(Alive_signal), Display/1, If/1
  If/1 -> Error_Counter/Action
  Error_Counter/1(Out1) -> Merge/1
  If1/1 -> Signal_Failure/Action
  If1/2 -> Signal_OK/Action
  Signal_Failure/1(Out1) -> Merge1/1
  Signal_OK/1(Out1) -> Merge1/2
  Merge1/1 -> Display2/1, Disconnect_Fail/1

== system Disconnections_ETR07/Subsystem/Others ==
  In1 : Inport
  Action Port : ActionPort  ActionType=else
  others : Outport
  wires:
  In1/1 -> others/1

== system Disconnections_ETR07/Subsystem/Others  ==
  In1 : Inport
  Action Port : ActionPort  ActionType=else
  others : Outport
  wires:
  In1/1 -> others/1

== system Disconnections_ETR07/Subsystem/Rigid Axle ==
  Action Port : ActionPort  ActionType=else
  Constant : Constant  Value=3
  3 : Outport
  wires:
  Constant/1 -> 3/1

== system Disconnections_ETR07/Subsystem/Steering TV 2017 without TC ==
  Action Port : ActionPort  ActionType=then
  Constant : Constant  Value=2
  2 : Outport
  wires:
  Constant/1 -> 2/1

== system Disconnections_ETR07/Subsystem/VDC 2018 Complete ==
  Action Port : ActionPort  ActionType=then
  Constant : Constant  Value=0
  0 : Outport
  wires:
  Constant/1 -> 0/1

== system Disconnections_ETR07/Subsystem/VDC without Longitudinal  ==
  Action Port : ActionPort  ActionType=then
  Constant : Constant
  1 : Outport
  wires:
  Constant/1 -> 1/1

== system Disconnections_ETR07/ECU Disconections/LifeCheck_ADCAN/CAN_OK ==
  Alive_signal : Inport
  Action Port : ActionPort  ActionType=else
  Constant : Constant  Value=0
  Data Store Write : DataStoreWrite  DataStoreName=Last_alive
  Out1 : Outport
  wires:
  Constant/1 -> Out1/1
  Alive_signal/1 -> Data Store Write/1

== system Disconnections_ETR07/ECU Disconections/LifeCheck_ADCAN/CAN_failure ==
  Action Port : ActionPort  ActionType=then
  Constant : Constant
  Out1 : Outport
  wires:
  Constant/1 -> Out1/1

== system Disconnections_ETR07/ECU Disconections/LifeCheck_AccFront/CAN_OK ==
  Alive_signal : Inport
  Action Port : ActionPort  ActionType=else
  Constant : Constant  Value=0
  Data Store Write : DataStoreWrite  DataStoreName=Last_alive
  Out1 : Outport
  wires:
  Constant/1 -> Out1/1
  Alive_signal/1 -> Data Store Write/1

== system Disconnections_ETR07/ECU Disconections/LifeCheck_AccFront/CAN_failure ==
  Action Port : ActionPort  ActionType=then
  Constant : Constant
  Out1 : Outport
  wires:
  Constant/1 -> Out1/1

== system Disconnections_ETR07/ECU Disconections/LifeCheck_AccRear/CAN_OK ==
  Alive_signal : Inport
  Action Port : ActionPort  ActionType=else
  Constant : Constant  Value=0
  Data Store Write : DataStoreWrite  DataStoreName=Last_alive
  Out1 : Outport
  wires:
  Constant/1 -> Out1/1
  Alive_signal/1 -> Data Store Write/1

== system Disconnections_ETR07/ECU Disconections/LifeCheck_AccRear/CAN_failure ==
  Action Port : ActionPort  ActionType=then
  Constant : Constant
  Out1 : Outport
  wires:
  Constant/1 -> Out1/1

== system Disconnections_ETR07/ECU Disconections/LifeCheck_BMS/CAN_OK ==
  Alive_signal : Inport
  Action Port : ActionPort  ActionType=else
  Constant : Constant  Value=0
  Data Store Write : DataStoreWrite  DataStoreName=Last_alive
  Out1 : Outport
  wires:
  Constant/1 -> Out1/1
  Alive_signal/1 -> Data Store Write/1

== system Disconnections_ETR07/ECU Disconections/LifeCheck_BMS/CAN_failure ==
  Action Port : ActionPort  ActionType=then
  Constant : Constant
  Out1 : Outport
  wires:
  Constant/1 -> Out1/1

== system Disconnections_ETR07/ECU Disconections/LifeCheck_Dash/CAN_OK ==
  Alive_signal : Inport
  Action Port : ActionPort  ActionType=else
  Constant : Constant  Value=0
  Data Store Write : DataStoreWrite  DataStoreName=Last_alive
  Out1 : Outport
  wires:
  Constant/1 -> Out1/1
  Alive_signal/1 -> Data Store Write/1

== system Disconnections_ETR07/ECU Disconections/LifeCheck_Dash/CAN_failure ==
  Action Port : ActionPort  ActionType=then
  Constant : Constant
  Out1 : Outport
  wires:
  Constant/1 -> Out1/1

== system Disconnections_ETR07/ECU Disconections/LifeCheck_Shutdown/CAN_OK ==
  Alive_signal : Inport
  Action Port : ActionPort  ActionType=else
  Constant : Constant  Value=0
  Data Store Write : DataStoreWrite  DataStoreName=Last_alive
  Out1 : Outport
  wires:
  Constant/1 -> Out1/1
  Alive_signal/1 -> Data Store Write/1

== system Disconnections_ETR07/ECU Disconections/LifeCheck_Shutdown/CAN_failure ==
  Action Port : ActionPort  ActionType=then
  Constant : Constant
  Out1 : Outport
  wires:
  Constant/1 -> Out1/1

== system Disconnections_ETR07/ECU Disconections/Life_check4/CAN_OK ==
  Alive_signal : Inport
  Action Port : ActionPort  ActionType=else
  Constant : Constant  Value=0
  Data Store Write : DataStoreWrite  DataStoreName=Last_alive
  Out1 : Outport
  wires:
  Constant/1 -> Out1/1
  Alive_signal/1 -> Data Store Write/1

== system Disconnections_ETR07/ECU Disconections/Life_check4/CAN_failure ==
  Action Port : ActionPort  ActionType=then
  Constant : Constant
  Out1 : Outport
  wires:
  Constant/1 -> Out1/1

== system Disconnections_ETR07/Gyro Disconnections (Noise)/Life_check6/CAN_OK ==
  Alive_signal : Inport
  Action Port : ActionPort  ActionType=else
  Constant : Constant  Value=0
  Data Store Write : DataStoreWrite  DataStoreName=Last_alive
  Out1 : Outport
  wires:
  Constant/1 -> Out1/1
  Alive_signal/1 -> Data Store Write/1

== system Disconnections_ETR07/Gyro Disconnections (Noise)/Life_check6/Error_Counter ==
  Action Port : ActionPort  ActionType=then
  Add : Sum
  Constant : Constant
  Data Store Read1 : DataStoreRead  DataStoreName=Tot_Errors
  Display3 : Display
  Out1 : Outport
  wires:
  Constant/1 -> Add/2
  Data Store Read1/1 -> Display3/1, Add/1
  Add/1 -> Out1/1

== system Disconnections_ETR07/Gyro Disconnections (Noise)/Life_check6/Signal_Failure ==
  Action Port : ActionPort  ActionType=then
  Constant : Constant
  Out1 : Outport
  wires:
  Constant/1 -> Out1/1

== system Disconnections_ETR07/Gyro Disconnections (Noise)/Life_check6/Signal_OK ==
  Action Port : ActionPort  ActionType=else
  Constant : Constant  Value=0
  Out1 : Outport
  wires:
  Constant/1 -> Out1/1

== system Disconnections_ETR07/Gyro Disconnections (Noise)/Life_check8/CAN_OK ==
  Alive_signal : Inport
  Action Port : ActionPort  ActionType=else
  Constant : Constant  Value=0
  Data Store Write : DataStoreWrite  DataStoreName=Last_alive
  Out1 : Outport
  wires:
  Constant/1 -> Out1/1
  Alive_signal/1 -> Data Store Write/1

== system Disconnections_ETR07/Gyro Disconnections (Noise)/Life_check8/Error_Counter ==
  Action Port : ActionPort  ActionType=then
  Add : Sum
  Constant : Constant
  Data Store Read1 : DataStoreRead  DataStoreName=Tot_Errors
  Display3 : Display
  Out1 : Outport
  wires:
  Constant/1 -> Add/2
  Data Store Read1/1 -> Display3/1, Add/1
  Add/1 -> Out1/1

== system Disconnections_ETR07/Gyro Disconnections (Noise)/Life_check8/Signal_Failure ==
  Action Port : ActionPort  ActionType=then
  Constant : Constant
  Out1 : Outport
  wires:
  Constant/1 -> Out1/1

== system Disconnections_ETR07/Gyro Disconnections (Noise)/Life_check8/Signal_OK ==
  Action Port : ActionPort  ActionType=else
  Constant : Constant  Value=0
  Out1 : Outport
  wires:
  Constant/1 -> Out1/1

== system Disconnections_ETR07/Pedal Box Disconnections (Noise)/Life_check1/CAN_OK ==
  Alive_signal : Inport
  Action Port : ActionPort  ActionType=else
  Constant : Constant  Value=0
  Data Store Write : DataStoreWrite  DataStoreName=Last_alive
  Out1 : Outport
  wires:
  Constant/1 -> Out1/1
  Alive_signal/1 -> Data Store Write/1

== system Disconnections_ETR07/Pedal Box Disconnections (Noise)/Life_check1/Error_Counter ==
  Action Port : ActionPort  ActionType=then
  Add : Sum
  Constant : Constant
  Data Store Read1 : DataStoreRead  DataStoreName=Tot_Errors
  Display3 : Display
  Out1 : Outport
  wires:
  Constant/1 -> Add/2
  Data Store Read1/1 -> Display3/1, Add/1
  Add/1 -> Out1/1

== system Disconnections_ETR07/Pedal Box Disconnections (Noise)/Life_check1/Signal_Failure ==
  Action Port : ActionPort  ActionType=then
  Constant : Constant
  Out1 : Outport
  wires:
  Constant/1 -> Out1/1

== system Disconnections_ETR07/Pedal Box Disconnections (Noise)/Life_check1/Signal_OK ==
  Action Port : ActionPort  ActionType=else
  Constant : Constant  Value=0
  Out1 : Outport
  wires:
  Constant/1 -> Out1/1

== system Disconnections_ETR07/Pedal Box Disconnections (Noise)/Life_check2/CAN_OK ==
  Alive_signal : Inport
  Action Port : ActionPort  ActionType=else
  Constant : Constant  Value=0
  Data Store Write : DataStoreWrite  DataStoreName=Last_alive
  Out1 : Outport
  wires:
  Constant/1 -> Out1/1
  Alive_signal/1 -> Data Store Write/1

== system Disconnections_ETR07/Pedal Box Disconnections (Noise)/Life_check2/Error_Counter ==
  Action Port : ActionPort  ActionType=then
  Add : Sum
  Constant : Constant
  Data Store Read1 : DataStoreRead  DataStoreName=Tot_Errors
  Display3 : Display
  Out1 : Outport
  wires:
  Constant/1 -> Add/2
  Data Store Read1/1 -> Display3/1, Add/1
  Add/1 -> Out1/1

== system Disconnections_ETR07/Pedal Box Disconnections (Noise)/Life_check2/Signal_Failure ==
  Action Port : ActionPort  ActionType=then
  Constant : Constant
  Out1 : Outport
  wires:
  Constant/1 -> Out1/1

== system Disconnections_ETR07/Pedal Box Disconnections (Noise)/Life_check2/Signal_OK ==
  Action Port : ActionPort  ActionType=else
  Constant : Constant  Value=0
  Out1 : Outport
  wires:
  Constant/1 -> Out1/1

== system Disconnections_ETR07/Pedal Box Disconnections (Noise)/Life_check3/CAN_OK ==
  Alive_signal : Inport
  Action Port : ActionPort  ActionType=else
  Constant : Constant  Value=0
  Data Store Write : DataStoreWrite  DataStoreName=Last_alive
  Out1 : Outport
  wires:
  Constant/1 -> Out1/1
  Alive_signal/1 -> Data Store Write/1

== system Disconnections_ETR07/Pedal Box Disconnections (Noise)/Life_check3/Error_Counter ==
  Action Port : ActionPort  ActionType=then
  Add : Sum
  Constant : Constant
  Data Store Read1 : DataStoreRead  DataStoreName=Tot_Errors
  Display3 : Display
  Out1 : Outport
  wires:
  Constant/1 -> Add/2
  Data Store Read1/1 -> Display3/1, Add/1
  Add/1 -> Out1/1

== system Disconnections_ETR07/Pedal Box Disconnections (Noise)/Life_check3/Signal_Failure ==
  Action Port : ActionPort  ActionType=then
  Constant : Constant
  Out1 : Outport
  wires:
  Constant/1 -> Out1/1

== system Disconnections_ETR07/Pedal Box Disconnections (Noise)/Life_check3/Signal_OK ==
  Action Port : ActionPort  ActionType=else
  Constant : Constant  Value=0
  Out1 : Outport
  wires:
  Constant/1 -> Out1/1
